simulink model "MIL4L3_SW6_V1_20220211"  (R2018b)
settings: Solver=FixedStepAuto  StartTime=0.0  StopTime=inf  FixedStep=0.001  RelTol=1e-3
PreLoadFcn:
  | A0_MILtest;
undefined symbols (not defined in the file or in its folder): Clb_ICADirect_LaneDisp_StateFive, Clb_ICADirect_LaneDisp_StateFour, Clb_ICADirect_LaneDisp_StateOne, Clb_ICADirect_LaneDisp_StateThree, Clb_ICADirect_LaneDisp_StateTwo, Clb_ICADirect_LaneDisp_StateZero, Clb_ICADirect_LaneDispSW, Clb_ICADirect_TrnLghtsCom_Switch, Clb_ICADirect_TrnLghtsCom_Value, Clb_ICADirect_TrnLghtsCrtl_Inhb, IMAP_Clb_ACU_Driver_Belt, IMAP_Clb_ACU_Driver_Belt_Over, IMAP_Clb_ACU_Passenger_Belt, IMAP_Clb_ACU_Passenger_Belt_Over, IMAP_Clb_ACU_RearLeft_Belt, IMAP_Clb_ACU_RearLeft_Belt_Over, IMAP_Clb_ACU_RearMiddle_Belt, IMAP_Clb_ACU_RearMiddle_Belt_Over, IMAP_Clb_ACU_RearRight_Belt, IMAP_Clb_ACU_RearRight_Belt_Over, IMAP_Clb_AEB_Switch, IMAP_Clb_AEB_Switch_Over, IMAP_Clb_ALC_TLC_Mode, IMAP_Clb_ALC_TLC_Mode_Over, IMAP_Clb_BCM_Battery_Voltage, IMAP_Clb_BCM_Battery_Voltage_Over, IMAP_Clb_BCM_BrakeLamp_State, IMAP_Clb_BCM_BrakeLamp_State_Over, IMAP_Clb_BCM_CHMSL_Status, IMAP_Clb_BCM_CHMSL_Status_Over, IMAP_Clb_BCM_Door_Lock_State, IMAP_Clb_BCM_Door_Lock_State_Over, IMAP_Clb_BCM_FrontWiper_State, IMAP_Clb_BCM_FrontWiper_State_Over, IMAP_Clb_BCM_FrontWiper_Switch, IMAP_Clb_BCM_FrontWiper_Switch_Over, IMAP_Clb_BCM_HazardLamp, IMAP_Clb_BCM_HazardLamp_Over, IMAP_Clb_BCM_HazardLamp_Switch, IMAP_Clb_BCM_HazardLamp_Switch_Over, IMAP_Clb_BCM_HighBeam_State, IMAP_Clb_BCM_HighBeam_State_Over, IMAP_Clb_BCM_Ignition_State, IMAP_Clb_BCM_Ignition_State_Over, IMAP_Clb_BCM_IHBC_Enabled, IMAP_Clb_BCM_IHBC_Enabled_Over, IMAP_Clb_BCM_Left_Light, IMAP_Clb_BCM_Left_Light_Over, IMAP_Clb_BCM_LeftTurn_Switch, IMAP_Clb_BCM_LeftTurn_Switch_Over, IMAP_Clb_BCM_LF_Door_State, IMAP_Clb_BCM_LF_Door_State_Over, IMAP_Clb_BCM_LowBeam_State, IMAP_Clb_BCM_LowBeam_State_Over, IMAP_Clb_BCM_LR_Door_State, IMAP_Clb_BCM_LR_Door_State_Over, IMAP_Clb_BCM_RF_Door_State, IMAP_Clb_BCM_RF_Door_State_Over, IMAP_Clb_BCM_Right_Light, IMAP_Clb_BCM_Right_Light_Over ... (+547)
libraries: CarMaker4SL x2153, simulink x292, dspstat3 x3, canmsglib x2, simulink_extras x1
(part 19 of 52)

== system MIL4L3_SW6_V1_20220211/CarMaker/VehicleControl/Traffic Attribution Define1/T17 ==
  Define CM Dict 0 : CarMaker4SL/Define CM Dict  xname=User.IO.Out.T17.ExistenceProbability  xmono=off  xtype=Double4  xdvaplace=IO_Out  xnstates=0  xfirststate=0  xinitial=0.95
  Define CM Dict 1 : CarMaker4SL/Define CM Dict  xname=User.IO.Out.T17.class  xmono=off  xtype=Double4  xdvaplace=IO_Out  xnstates=0  xfirststate=0  xinitial=1
  Define CM Dict 2 : CarMaker4SL/Define CM Dict  xname=User.IO.Out.T17.ObjectInfo  xmono=off  xtype=Double4  xdvaplace=IO_Out  xnstates=0  xfirststate=0  xinitial=2
  Define CM Dict 3 : CarMaker4SL/Define CM Dict  xname=User.IO.Out.T17.ClassHighestProb  xmono=off  xtype=Double4  xdvaplace=IO_Out  xnstates=0  xfirststate=0  xinitial=2
  Define CM Dict 4 : CarMaker4SL/Define CM Dict  xname=User.IO.Out.T17.status  xmono=off  xtype=Double4  xdvaplace=IO_Out  xnstates=0  xfirststate=0  xinitial=0
  Define CM Dict 5 : CarMaker4SL/Define CM Dict  xname=User.IO.Out.T17.probility  xmono=off  xtype=Double4  xdvaplace=IO_Out  xnstates=0  xfirststate=0  xinitial=0.9
  Define CM Dict 6 : CarMaker4SL/Define CM Dict  xname=User.IO.Out.T17.power  xmono=off  xtype=Double4  xdvaplace=IO_Out  xnstates=0  xfirststate=0  xinitial=90
  Define CM Dict 7 : CarMaker4SL/Define CM Dict  xname=User.IO.Out.T17.Turn_signal  xmono=off  xtype=Double4  xdvaplace=IO_Out  xnstates=0  xfirststate=0  xinitial=0
  Define CM Dict 8 : CarMaker4SL/Define CM Dict  xname=User.IO.Out.T17.BrakeLight  xmono=off  xtype=Double4  xdvaplace=IO_Out  xnstates=0  xfirststate=0  xinitial=0
  Define CM Dict5 : CarMaker4SL/Define CM Dict  xname=User.IO.Out.T17.longdistance  xmono=off  xtype=Double4  xdvaplace=None  xnstates=0  xfirststate=0  xinitial=0
  Define CM Dict6 : CarMaker4SL/Define CM Dict  xname=User.IO.Out.T17.RelVxValid  xmono=off  xtype=Double4  xdvaplace=None  xnstates=0  xfirststate=0  xinitial=1
  Define CM Dict7 : CarMaker4SL/Define CM Dict  xname=User.IO.Out.T17.RelVyValid  xmono=off  xtype=Double4  xdvaplace=None  xnstates=0  xfirststate=0  xinitial=1
  Define CM Dict8 : CarMaker4SL/Define CM Dict  xname=User.IO.Out.T17.TypeProb  xmono=off  xtype=Double4  xdvaplace=None  xnstates=0  xfirststate=0  xinitial=1
  Define CM Dict9 : CarMaker4SL/Define CM Dict  xname=User.IO.Out.T17.Measured  xmono=off  xtype=Double4  xdvaplace=None  xnstates=0  xfirststate=0  xinitial=2

== system MIL4L3_SW6_V1_20220211/CarMaker/VehicleControl/Traffic Attribution Define1/T18 ==
  Define CM Dict 0 : CarMaker4SL/Define CM Dict  xname=User.IO.Out.T18.ExistenceProbability  xmono=off  xtype=Double4  xdvaplace=IO_Out  xnstates=0  xfirststate=0  xinitial=0.95
  Define CM Dict 1 : CarMaker4SL/Define CM Dict  xname=User.IO.Out.T18.class  xmono=off  xtype=Double4  xdvaplace=IO_Out  xnstates=0  xfirststate=0  xinitial=1
  Define CM Dict 2 : CarMaker4SL/Define CM Dict  xname=User.IO.Out.T18.ObjectInfo  xmono=off  xtype=Double4  xdvaplace=IO_Out  xnstates=0  xfirststate=0  xinitial=2
  Define CM Dict 3 : CarMaker4SL/Define CM Dict  xname=User.IO.Out.T18.ClassHighestProb  xmono=off  xtype=Double4  xdvaplace=IO_Out  xnstates=0  xfirststate=0  xinitial=2
  Define CM Dict 4 : CarMaker4SL/Define CM Dict  xname=User.IO.Out.T18.status  xmono=off  xtype=Double4  xdvaplace=IO_Out  xnstates=0  xfirststate=0  xinitial=0
  Define CM Dict 5 : CarMaker4SL/Define CM Dict  xname=User.IO.Out.T18.probility  xmono=off  xtype=Double4  xdvaplace=IO_Out  xnstates=0  xfirststate=0  xinitial=0.9
  Define CM Dict 6 : CarMaker4SL/Define CM Dict  xname=User.IO.Out.T18.power  xmono=off  xtype=Double4  xdvaplace=IO_Out  xnstates=0  xfirststate=0  xinitial=90
  Define CM Dict 7 : CarMaker4SL/Define CM Dict  xname=User.IO.Out.T18.Turn_signal  xmono=off  xtype=Double4  xdvaplace=IO_Out  xnstates=0  xfirststate=0  xinitial=0
  Define CM Dict 8 : CarMaker4SL/Define CM Dict  xname=User.IO.Out.T18.BrakeLight  xmono=off  xtype=Double4  xdvaplace=IO_Out  xnstates=0  xfirststate=0  xinitial=0
  Define CM Dict5 : CarMaker4SL/Define CM Dict  xname=User.IO.Out.T18.longdistance  xmono=off  xtype=Double4  xdvaplace=None  xnstates=0  xfirststate=0  xinitial=0
  Define CM Dict6 : CarMaker4SL/Define CM Dict  xname=User.IO.Out.T18.RelVxValid  xmono=off  xtype=Double4  xdvaplace=None  xnstates=0  xfirststate=0  xinitial=1
  Define CM Dict7 : CarMaker4SL/Define CM Dict  xname=User.IO.Out.T18.RelVyValid  xmono=off  xtype=Double4  xdvaplace=None  xnstates=0  xfirststate=0  xinitial=1
  Define CM Dict8 : CarMaker4SL/Define CM Dict  xname=User.IO.Out.T18.TypeProb  xmono=off  xtype=Double4  xdvaplace=None  xnstates=0  xfirststate=0  xinitial=1
  Define CM Dict9 : CarMaker4SL/Define CM Dict  xname=User.IO.Out.T18.Measured  xmono=off  xtype=Double4  xdvaplace=None  xnstates=0  xfirststate=0  xinitial=2

== system MIL4L3_SW6_V1_20220211/CarMaker/VehicleControl/Traffic Attribution Define1/T19 ==
  Define CM Dict 0 : CarMaker4SL/Define CM Dict  xname=User.IO.Out.T19.ExistenceProbability  xmono=off  xtype=Double4  xdvaplace=IO_Out  xnstates=0  xfirststate=0  xinitial=0.95
  Define CM Dict 1 : CarMaker4SL/Define CM Dict  xname=User.IO.Out.T19.class  xmono=off  xtype=Double4  xdvaplace=IO_Out  xnstates=0  xfirststate=0  xinitial=1
  Define CM Dict 2 : CarMaker4SL/Define CM Dict  xname=User.IO.Out.T19.ObjectInfo  xmono=off  xtype=Double4  xdvaplace=IO_Out  xnstates=0  xfirststate=0  xinitial=2
  Define CM Dict 3 : CarMaker4SL/Define CM Dict  xname=User.IO.Out.T19.ClassHighestProb  xmono=off  xtype=Double4  xdvaplace=IO_Out  xnstates=0  xfirststate=0  xinitial=2
  Define CM Dict 4 : CarMaker4SL/Define CM Dict  xname=User.IO.Out.T19.status  xmono=off  xtype=Double4  xdvaplace=IO_Out  xnstates=0  xfirststate=0  xinitial=0
  Define CM Dict 5 : CarMaker4SL/Define CM Dict  xname=User.IO.Out.T19.probility  xmono=off  xtype=Double4  xdvaplace=IO_Out  xnstates=0  xfirststate=0  xinitial=0.9
  Define CM Dict 6 : CarMaker4SL/Define CM Dict  xname=User.IO.Out.T19.power  xmono=off  xtype=Double4  xdvaplace=IO_Out  xnstates=0  xfirststate=0  xinitial=90
  Define CM Dict 7 : CarMaker4SL/Define CM Dict  xname=User.IO.Out.T19.Turn_signal  xmono=off  xtype=Double4  xdvaplace=IO_Out  xnstates=0  xfirststate=0  xinitial=0
  Define CM Dict 8 : CarMaker4SL/Define CM Dict  xname=User.IO.Out.T19.BrakeLight  xmono=off  xtype=Double4  xdvaplace=IO_Out  xnstates=0  xfirststate=0  xinitial=0
  Define CM Dict5 : CarMaker4SL/Define CM Dict  xname=User.IO.Out.T19.longdistance  xmono=off  xtype=Double4  xdvaplace=None  xnstates=0  xfirststate=0  xinitial=0
  Define CM Dict6 : CarMaker4SL/Define CM Dict  xname=User.IO.Out.T19.RelVxValid  xmono=off  xtype=Double4  xdvaplace=None  xnstates=0  xfirststate=0  xinitial=1
  Define CM Dict7 : CarMaker4SL/Define CM Dict  xname=User.IO.Out.T19.RelVyValid  xmono=off  xtype=Double4  xdvaplace=None  xnstates=0  xfirststate=0  xinitial=1
  Define CM Dict8 : CarMaker4SL/Define CM Dict  xname=User.IO.Out.T19.TypeProb  xmono=off  xtype=Double4  xdvaplace=None  xnstates=0  xfirststate=0  xinitial=1
  Define CM Dict9 : CarMaker4SL/Define CM Dict  xname=User.IO.Out.T19.Measured  xmono=off  xtype=Double4  xdvaplace=None  xnstates=0  xfirststate=0  xinitial=2

== system MIL4L3_SW6_V1_20220211/CarMaker/VehicleControl/Traffic Attribution Define1/T20 ==
  Define CM Dict 0 : CarMaker4SL/Define CM Dict  xname=User.IO.Out.T20.ExistenceProbability  xmono=off  xtype=Double4  xdvaplace=IO_Out  xnstates=0  xfirststate=0  xinitial=0.95
  Define CM Dict 1 : CarMaker4SL/Define CM Dict  xname=User.IO.Out.T20.class  xmono=off  xtype=Double4  xdvaplace=IO_Out  xnstates=0  xfirststate=0  xinitial=1
  Define CM Dict 2 : CarMaker4SL/Define CM Dict  xname=User.IO.Out.T20.ObjectInfo  xmono=off  xtype=Double4  xdvaplace=IO_Out  xnstates=0  xfirststate=0  xinitial=2
  Define CM Dict 3 : CarMaker4SL/Define CM Dict  xname=User.IO.Out.T20.ClassHighestProb  xmono=off  xtype=Double4  xdvaplace=IO_Out  xnstates=0  xfirststate=0  xinitial=2
  Define CM Dict 4 : CarMaker4SL/Define CM Dict  xname=User.IO.Out.T20.status  xmono=off  xtype=Double4  xdvaplace=IO_Out  xnstates=0  xfirststate=0  xinitial=0
  Define CM Dict 5 : CarMaker4SL/Define CM Dict  xname=User.IO.Out.T20.probility  xmono=off  xtype=Double4  xdvaplace=IO_Out  xnstates=0  xfirststate=0  xinitial=0.9
  Define CM Dict 6 : CarMaker4SL/Define CM Dict  xname=User.IO.Out.T20.power  xmono=off  xtype=Double4  xdvaplace=IO_Out  xnstates=0  xfirststate=0  xinitial=90
  Define CM Dict 7 : CarMaker4SL/Define CM Dict  xname=User.IO.Out.T20.Turn_signal  xmono=off  xtype=Double4  xdvaplace=IO_Out  xnstates=0  xfirststate=0  xinitial=0
  Define CM Dict 8 : CarMaker4SL/Define CM Dict  xname=User.IO.Out.T20.BrakeLight  xmono=off  xtype=Double4  xdvaplace=IO_Out  xnstates=0  xfirststate=0  xinitial=0
  Define CM Dict5 : CarMaker4SL/Define CM Dict  xname=User.IO.Out.T20.longdistance  xmono=off  xtype=Double4  xdvaplace=None  xnstates=0  xfirststate=0  xinitial=0
  Define CM Dict6 : CarMaker4SL/Define CM Dict  xname=User.IO.Out.T20.RelVxValid  xmono=off  xtype=Double4  xdvaplace=None  xnstates=0  xfirststate=0  xinitial=1
  Define CM Dict7 : CarMaker4SL/Define CM Dict  xname=User.IO.Out.T20.RelVyValid  xmono=off  xtype=Double4  xdvaplace=None  xnstates=0  xfirststate=0  xinitial=1
  Define CM Dict8 : CarMaker4SL/Define CM Dict  xname=User.IO.Out.T20.TypeProb  xmono=off  xtype=Double4  xdvaplace=None  xnstates=0  xfirststate=0  xinitial=1
  Define CM Dict9 : CarMaker4SL/Define CM Dict  xname=User.IO.Out.T20.Measured  xmono=off  xtype=Double4  xdvaplace=None  xnstates=0  xfirststate=0  xinitial=2

== system MIL4L3_SW6_V1_20220211/CarMaker/VehicleControl/Traffic Attribution Define1/T21 ==
  Define CM Dict 0 : CarMaker4SL/Define CM Dict  xname=User.IO.Out.T21.ExistenceProbability  xmono=off  xtype=Double4  xdvaplace=IO_Out  xnstates=0  xfirststate=0  xinitial=0.95
  Define CM Dict 1 : CarMaker4SL/Define CM Dict  xname=User.IO.Out.T21.class  xmono=off  xtype=Double4  xdvaplace=IO_Out  xnstates=0  xfirststate=0  xinitial=1
  Define CM Dict 2 : CarMaker4SL/Define CM Dict  xname=User.IO.Out.T21.ObjectInfo  xmono=off  xtype=Double4  xdvaplace=IO_Out  xnstates=0  xfirststate=0  xinitial=2
  Define CM Dict 3 : CarMaker4SL/Define CM Dict  xname=User.IO.Out.T21.ClassHighestProb  xmono=off  xtype=Double4  xdvaplace=IO_Out  xnstates=0  xfirststate=0  xinitial=2
  Define CM Dict 4 : CarMaker4SL/Define CM Dict  xname=User.IO.Out.T21.status  xmono=off  xtype=Double4  xdvaplace=IO_Out  xnstates=0  xfirststate=0  xinitial=0
  Define CM Dict 5 : CarMaker4SL/Define CM Dict  xname=User.IO.Out.T21.probility  xmono=off  xtype=Double4  xdvaplace=IO_Out  xnstates=0  xfirststate=0  xinitial=0.9
  Define CM Dict 6 : CarMaker4SL/Define CM Dict  xname=User.IO.Out.T21.power  xmono=off  xtype=Double4  xdvaplace=IO_Out  xnstates=0  xfirststate=0  xinitial=90
  Define CM Dict 7 : CarMaker4SL/Define CM Dict  xname=User.IO.Out.T21.Turn_signal  xmono=off  xtype=Double4  xdvaplace=IO_Out  xnstates=0  xfirststate=0  xinitial=0
  Define CM Dict 8 : CarMaker4SL/Define CM Dict  xname=User.IO.Out.T21.BrakeLight  xmono=off  xtype=Double4  xdvaplace=IO_Out  xnstates=0  xfirststate=0  xinitial=0
  Define CM Dict5 : CarMaker4SL/Define CM Dict  xname=User.IO.Out.T21.longdistance  xmono=off  xtype=Double4  xdvaplace=None  xnstates=0  xfirststate=0  xinitial=0
  Define CM Dict6 : CarMaker4SL/Define CM Dict  xname=User.IO.Out.T21.RelVxValid  xmono=off  xtype=Double4  xdvaplace=None  xnstates=0  xfirststate=0  xinitial=1
  Define CM Dict7 : CarMaker4SL/Define CM Dict  xname=User.IO.Out.T21.RelVyValid  xmono=off  xtype=Double4  xdvaplace=None  xnstates=0  xfirststate=0  xinitial=1
  Define CM Dict8 : CarMaker4SL/Define CM Dict  xname=User.IO.Out.T21.TypeProb  xmono=off  xtype=Double4  xdvaplace=None  xnstates=0  xfirststate=0  xinitial=1
  Define CM Dict9 : CarMaker4SL/Define CM Dict  xname=User.IO.Out.T21.Measured  xmono=off  xtype=Double4  xdvaplace=None  xnstates=0  xfirststate=0  xinitial=2

== system MIL4L3_SW6_V1_20220211/CarMaker/VehicleControl/Traffic Attribution Define1/T22 ==
  Define CM Dict 0 : CarMaker4SL/Define CM Dict  xname=User.IO.Out.T22.ExistenceProbability  xmono=off  xtype=Double4  xdvaplace=IO_Out  xnstates=0  xfirststate=0  xinitial=0.95
  Define CM Dict 1 : CarMaker4SL/Define CM Dict  xname=User.IO.Out.T22.class  xmono=off  xtype=Double4  xdvaplace=IO_Out  xnstates=0  xfirststate=0  xinitial=1
  Define CM Dict 2 : CarMaker4SL/Define CM Dict  xname=User.IO.Out.T22.ObjectInfo  xmono=off  xtype=Double4  xdvaplace=IO_Out  xnstates=0  xfirststate=0  xinitial=2
  Define CM Dict 3 : CarMaker4SL/Define CM Dict  xname=User.IO.Out.T22.ClassHighestProb  xmono=off  xtype=Double4  xdvaplace=IO_Out  xnstates=0  xfirststate=0  xinitial=2
  Define CM Dict 4 : CarMaker4SL/Define CM Dict  xname=User.IO.Out.T22.status  xmono=off  xtype=Double4  xdvaplace=IO_Out  xnstates=0  xfirststate=0  xinitial=0
  Define CM Dict 5 : CarMaker4SL/Define CM Dict  xname=User.IO.Out.T22.probility  xmono=off  xtype=Double4  xdvaplace=IO_Out  xnstates=0  xfirststate=0  xinitial=0.9
  Define CM Dict 6 : CarMaker4SL/Define CM Dict  xname=User.IO.Out.T22.power  xmono=off  xtype=Double4  xdvaplace=IO_Out  xnstates=0  xfirststate=0  xinitial=90
  Define CM Dict 7 : CarMaker4SL/Define CM Dict  xname=User.IO.Out.T22.Turn_signal  xmono=off  xtype=Double4  xdvaplace=IO_Out  xnstates=0  xfirststate=0  xinitial=0
  Define CM Dict 8 : CarMaker4SL/Define CM Dict  xname=User.IO.Out.T22.BrakeLight  xmono=off  xtype=Double4  xdvaplace=IO_Out  xnstates=0  xfirststate=0  xinitial=0
  Define CM Dict5 : CarMaker4SL/Define CM Dict  xname=User.IO.Out.T22.longdistance  xmono=off  xtype=Double4  xdvaplace=None  xnstates=0  xfirststate=0  xinitial=0
  Define CM Dict6 : CarMaker4SL/Define CM Dict  xname=User.IO.Out.T22.RelVxValid  xmono=off  xtype=Double4  xdvaplace=None  xnstates=0  xfirststate=0  xinitial=1
  Define CM Dict7 : CarMaker4SL/Define CM Dict  xname=User.IO.Out.T22.RelVyValid  xmono=off  xtype=Double4  xdvaplace=None  xnstates=0  xfirststate=0  xinitial=1
  Define CM Dict8 : CarMaker4SL/Define CM Dict  xname=User.IO.Out.T22.TypeProb  xmono=off  xtype=Double4  xdvaplace=None  xnstates=0  xfirststate=0  xinitial=1
  Define CM Dict9 : CarMaker4SL/Define CM Dict  xname=User.IO.Out.T22.Measured  xmono=off  xtype=Double4  xdvaplace=None  xnstates=0  xfirststate=0  xinitial=2

== system MIL4L3_SW6_V1_20220211/CarMaker/VehicleControl/Traffic Attribution Define1/T23 ==
  Define CM Dict 0 : CarMaker4SL/Define CM Dict  xname=User.IO.Out.T23.ExistenceProbability  xmono=off  xtype=Double4  xdvaplace=IO_Out  xnstates=0  xfirststate=0  xinitial=0.95
  Define CM Dict 1 : CarMaker4SL/Define CM Dict  xname=User.IO.Out.T23.class  xmono=off  xtype=Double4  xdvaplace=IO_Out  xnstates=0  xfirststate=0  xinitial=1
  Define CM Dict 2 : CarMaker4SL/Define CM Dict  xname=User.IO.Out.T23.ObjectInfo  xmono=off  xtype=Double4  xdvaplace=IO_Out  xnstates=0  xfirststate=0  xinitial=2
  Define CM Dict 3 : CarMaker4SL/Define CM Dict  xname=User.IO.Out.T23.ClassHighestProb  xmono=off  xtype=Double4  xdvaplace=IO_Out  xnstates=0  xfirststate=0  xinitial=2
  Define CM Dict 4 : CarMaker4SL/Define CM Dict  xname=User.IO.Out.T23.status  xmono=off  xtype=Double4  xdvaplace=IO_Out  xnstates=0  xfirststate=0  xinitial=0
  Define CM Dict 5 : CarMaker4SL/Define CM Dict  xname=User.IO.Out.T23.probility  xmono=off  xtype=Double4  xdvaplace=IO_Out  xnstates=0  xfirststate=0  xinitial=0.9
  Define CM Dict 6 : CarMaker4SL/Define CM Dict  xname=User.IO.Out.T23.power  xmono=off  xtype=Double4  xdvaplace=IO_Out  xnstates=0  xfirststate=0  xinitial=90
  Define CM Dict 7 : CarMaker4SL/Define CM Dict  xname=User.IO.Out.T23.Turn_signal  xmono=off  xtype=Double4  xdvaplace=IO_Out  xnstates=0  xfirststate=0  xinitial=0
  Define CM Dict 8 : CarMaker4SL/Define CM Dict  xname=User.IO.Out.T23.BrakeLight  xmono=off  xtype=Double4  xdvaplace=IO_Out  xnstates=0  xfirststate=0  xinitial=0
  Define CM Dict5 : CarMaker4SL/Define CM Dict  xname=User.IO.Out.T23.longdistance  xmono=off  xtype=Double4  xdvaplace=None  xnstates=0  xfirststate=0  xinitial=0
  Define CM Dict6 : CarMaker4SL/Define CM Dict  xname=User.IO.Out.T23.RelVxValid  xmono=off  xtype=Double4  xdvaplace=None  xnstates=0  xfirststate=0  xinitial=1
  Define CM Dict7 : CarMaker4SL/Define CM Dict  xname=User.IO.Out.T23.RelVyValid  xmono=off  xtype=Double4  xdvaplace=None  xnstates=0  xfirststate=0  xinitial=1
  Define CM Dict8 : CarMaker4SL/Define CM Dict  xname=User.IO.Out.T23.TypeProb  xmono=off  xtype=Double4  xdvaplace=None  xnstates=0  xfirststate=0  xinitial=1
  Define CM Dict9 : CarMaker4SL/Define CM Dict  xname=User.IO.Out.T23.Measured  xmono=off  xtype=Double4  xdvaplace=None  xnstates=0  xfirststate=0  xinitial=2

== system MIL4L3_SW6_V1_20220211/CarMaker/VehicleControl/User.IO.Out/ActuatorStatus2Ctrl ==
  BusCreator : BusCreator  Inputs=38
  Read CM Dict : CarMaker4SL/Read CM Dict  xname=User.IO.Out.EPS_LKAState  xsync=off
  Read CM Dict1 : CarMaker4SL/Read CM Dict  xname=User.IO.Out.EPSErrSt  xsync=off
  Read CM Dict10 : CarMaker4SL/Read CM Dict  xname=User.IO.Out.BCM_RRDoorSt  xsync=off
  Read CM Dict11 : CarMaker4SL/Read CM Dict  xname=User.IO.Out.BCM_LRDoorSt  xsync=off
  Read CM Dict12 : CarMaker4SL/Read CM Dict  xname=User.IO.Out.BCM_DoorLockSt  xsync=off
  Read CM Dict13 : CarMaker4SL/Read CM Dict  xname=User.IO.Out.EMS_Status_ACC  xsync=off
  Read CM Dict14 : CarMaker4SL/Read CM Dict  xname=User.IO.Out.SCC_LeftSwSig  xsync=off
  Read CM Dict15 : CarMaker4SL/Read CM Dict  xname=User.IO.Out.SCC_RightSwSig  xsync=off
  Read CM Dict16 : CarMaker4SL/Read CM Dict  xname=User.IO.Out.GW_EMS_AccPedFlt  xsync=off
  Read CM Dict17 : CarMaker4SL/Read CM Dict  xname=User.IO.Out.BCM_IgnitionSt  xsync=off
  Read CM Dict18 : CarMaker4SL/Read CM Dict  xname=User.IO.Out.EMS_AccPedalR  xsync=off
  Read CM Dict19 : CarMaker4SL/Read CM Dict  xname=User.IO.Out.GW_EMS_AccPedal  xsync=off
  Read CM Dict2 : CarMaker4SL/Read CM Dict  xname=User.IO.Out.BCM_HazardLampSt  xsync=off
  Read CM Dict20 : CarMaker4SL/Read CM Dict  xname=User.IO.Out.ACU_DriverBelt  xsync=off
  Read CM Dict21 : CarMaker4SL/Read CM Dict  xname=User.IO.Out.Brake_pedalFault  xsync=off
  Read CM Dict22 : CarMaker4SL/Read CM Dict  xname=User.IO.Out.GW_TCU_ATFailure  xsync=off
  Read CM Dict23 : CarMaker4SL/Read CM Dict  xname=User.IO.Out.ESC_ESCOFF  xsync=off
  Read CM Dict24 : CarMaker4SL/Read CM Dict  xname=User.IO.Out.GW_Speed_Lim_On  xsync=off
  Read CM Dict25 : CarMaker4SL/Read CM Dict  xname=User.IO.Out.BCM_FrontWiperSt  xsync=off
  Read CM Dict26 : CarMaker4SL/Read CM Dict  xname=User.IO.Out.ACU_PassengerBelt  xsync=off
  Read CM Dict27 : CarMaker4SL/Read CM Dict  xname=User.IO.Out.GW_EMS_EngStatus  xsync=off
  Read CM Dict28 : CarMaker4SL/Read CM Dict  xname=User.IO.Out.ESC_AEB_Status  xsync=off
  Read CM Dict29 : CarMaker4SL/Read CM Dict  xname=User.IO.Out.ESC_AEB_Available  xsync=off
  Read CM Dict3 : CarMaker4SL/Read CM Dict  xname=User.IO.Out.BCM_LetfligthSt  xsync=off
  Read CM Dict30 : CarMaker4SL/Read CM Dict  xname=User.IO.Out.ESC_ACC_Status  xsync=off
  Read CM Dict31 : CarMaker4SL/Read CM Dict  xname=User.IO.Out.ESC_ACC_Available  xsync=off
  Read CM Dict32 : CarMaker4SL/Read CM Dict  xname=User.IO.Out.EMS_ACCctlAvail  xsync=off
  Read CM Dict33 : CarMaker4SL/Read CM Dict  xname=User.IO.Out.EMS_ACC_Ihibited  xsync=off
  Read CM Dict34 : CarMaker4SL/Read CM Dict  xname=User.IO.Out.EPB_EPBStatus  xsync=off
  Read CM Dict35 : CarMaker4SL/Read CM Dict  xname=User.IO.Out.EPS_SteerHoldSt  xsync=off
  Read CM Dict36 : CarMaker4SL/Read CM Dict  xname=User.IO.Out.BCM_BattVolt  xsync=off
  Read CM Dict37 : CarMaker4SL/Read CM Dict  xname=User.IO.Out.ICAD_DecionState  xsync=off
  Read CM Dict4 : CarMaker4SL/Read CM Dict  xname=User.IO.Out.BCM_RightligthSt  xsync=off
  Read CM Dict5 : CarMaker4SL/Read CM Dict  xname=User.IO.Out.ESC_BLRequest  xsync=off
  Read CM Dict6 : CarMaker4SL/Read CM Dict  xname=User.IO.Out.BCM_Openingstates  xsync=off
  Read CM Dict7 : CarMaker4SL/Read CM Dict  xname=User.IO.Out.BCM_TrunkSt  xsync=off
  Read CM Dict8 : CarMaker4SL/Read CM Dict  xname=User.IO.Out.BCM_LFDoorSt  xsync=off
  Read CM Dict9 : CarMaker4SL/Read CM Dict  xname=User.IO.Out.BCM_RFDoorSt  xsync=off
  tag scope: ActuatorStatus2Ctrl=global
  wires:
  Read CM Dict6/1 -> BusCreator/7  "User.IO.Out.BCM_Openingstates"
  Read CM Dict7/1 -> BusCreator/8  "User.IO.Out.BCM_TrunkSt"
  Read CM Dict8/1 -> BusCreator/9  "User.IO.Out.BCM_LFDoorSt"
  Read CM Dict9/1 -> BusCreator/10  "User.IO.Out.BCM_RFDoorSt"
  Read CM Dict10/1 -> BusCreator/11  "User.IO.Out.BCM_RRDoorSt"
  Read CM Dict11/1 -> BusCreator/12  "User.IO.Out.BCM_LRDoorSt"
  Read CM Dict4/1 -> BusCreator/5  "User.IO.Out.BCM_RightligthSt"
  Read CM Dict5/1 -> BusCreator/6  "User.IO.Out.ESC_BLRequest"
  Read CM Dict14/1 -> BusCreator/13  "User.IO.Out.SCC_LeftSwSig"
  Read CM Dict15/1 -> BusCreator/14  "User.IO.Out.SCC_RightSwSig"
  Read CM Dict/1 -> BusCreator/1  "User.IO.Out.EPS_LKAState"
  Read CM Dict1/1 -> BusCreator/2  "User.IO.Out.EPSErrSt"
  Read CM Dict2/1 -> BusCreator/3  "User.IO.Out.BCM_HazardLampSt"
  Read CM Dict3/1 -> BusCreator/4  "User.IO.Out.BCM_LetfligthSt"
  Read CM Dict12/1 -> BusCreator/15  "User.IO.Out.BCM_DoorLockSt"
  Read CM Dict13/1 -> BusCreator/16  "User.IO.Out.EMS_Status_ACC"
  Read CM Dict18/1 -> BusCreator/17  "User.IO.Out.EMS_AccPedalR"
  Read CM Dict19/1 -> BusCreator/18  "User.IO.Out.GW_EMS_AccPedal"
  Read CM Dict16/1 -> BusCreator/19  "User.IO.Out.GW_EMS_AccPedFlt"
  Read CM Dict17/1 -> BusCreator/20  "User.IO.Out.BCM_IgnitionSt"
  Read CM Dict20/1 -> BusCreator/21  "User.IO.Out.ACU_DriverBelt"
  Read CM Dict23/1 -> BusCreator/22  "User.IO.Out.ESC_ESCOFF"
  Read CM Dict24/1 -> BusCreator/23  "User.IO.Out.GW_Speed_Lim_On"
  Read CM Dict21/1 -> BusCreator/24  "User.IO.Out.Brake_pedalFault"
  Read CM Dict22/1 -> BusCreator/25  "User.IO.Out.GW_TCU_ATFailure"
  Read CM Dict29/1 -> BusCreator/28  "User.IO.Out.ESC_AEB_Available"
  Read CM Dict30/1 -> BusCreator/29  "User.IO.Out.ESC_ACC_Status"
  Read CM Dict31/1 -> BusCreator/30  "User.IO.Out.ESC_ACC_Available"
  Read CM Dict26/1 -> BusCreator/32  "User.IO.Out.ACU_PassengerBelt"
  Read CM Dict32/1 -> BusCreator/33  "User.IO.Out.EMS_ACCctlAvail"
  Read CM Dict33/1 -> BusCreator/34  "User.IO.Out.EMS_ACC_Ihibited"
  Read CM Dict27/1 -> BusCreator/26  "User.IO.Out.GW_EMS_EngStatus"
  Read CM Dict28/1 -> BusCreator/27  "User.IO.Out.ESC_AEB_Status"
  Read CM Dict25/1 -> BusCreator/31  "User.IO.Out.BCM_FrontWiperSt"
  Read CM Dict35/1 -> BusCreator/36  "User.IO.Out.EPS_SteerHoldSt"
  Read CM Dict36/1 -> BusCreator/37  "User.IO.Out.BCM_BattVolt"
  Read CM Dict34/1 -> BusCreator/35  "User.IO.Out.EPB_EPBStatus"
  Read CM Dict37/1 -> BusCreator/38  "User.IO.Out.ICAD_DecionState"
  BusCreator/1 -> [ActuatorStatus2Ctrl]

== system MIL4L3_SW6_V1_20220211/CarMaker/VehicleControl/User.IO.Out/MP5_Cmd2Ctrl ==
  BusCreator : BusCreator  Inputs=27
  Read CM Dict : CarMaker4SL/Read CM Dict  xname=User.IO.Out.Mp5_LKA_main_SW  xsync=off
  Read CM Dict1 : CarMaker4SL/Read CM Dict  xname=User.IO.Out.Mp5_LKA_Mode  xsync=off
  Read CM Dict10 : CarMaker4SL/Read CM Dict  xname=User.IO.Out.MP5_ALCTLC_Mode  xsync=off
  Read CM Dict11 : CarMaker4SL/Read CM Dict  xname=User.IO.Out.Mp5_ESA_Cfg  xsync=off
  Read CM Dict12 : CarMaker4SL/Read CM Dict  xname=User.IO.Out.Mp5_ELK_Cfg  xsync=off
  Read CM Dict13 : CarMaker4SL/Read CM Dict  xname=User.IO.Out.AutoParkingCmd  xsync=off
  Read CM Dict14 : CarMaker4SL/Read CM Dict  xname=User.IO.Out.PEPS_RKECommand  xsync=off
  Read CM Dict15 : CarMaker4SL/Read CM Dict  xname=User.IO.Out.MP5_BSD_LCW_ACT  xsync=off
  Read CM Dict16 : CarMaker4SL/Read CM Dict  xname=User.IO.Out.MP5_RCTA_ACT  xsync=off
  Read CM Dict17 : CarMaker4SL/Read CM Dict  xname=User.IO.Out.MP5_DOW_ACT  xsync=off
  Read CM Dict18 : CarMaker4SL/Read CM Dict  xname=User.IO.Out.JaBrakConf  xsync=off
  Read CM Dict19 : CarMaker4SL/Read CM Dict  xname=User.IO.Out.JaAlertConf  xsync=off
  Read CM Dict2 : CarMaker4SL/Read CM Dict  xname=User.IO.Out.MP5_AEBSwitch  xsync=off
  Read CM Dict20 : CarMaker4SL/Read CM Dict  xname=User.IO.Out.JaAlertSens  xsync=off
  Read CM Dict21 : CarMaker4SL/Read CM Dict  xname=User.IO.Out.LFConf  xsync=off
  Read CM Dict22 : CarMaker4SL/Read CM Dict  xname=User.IO.Out.MP5_FCTA_ACT  xsync=off
  Read CM Dict23 : CarMaker4SL/Read CM Dict  xname=User.IO.Out.ICAConf  xsync=off
  Read CM Dict24 : CarMaker4SL/Read CM Dict  xname=User.IO.Out.AlcSens  xsync=off
  Read CM Dict25 : CarMaker4SL/Read CM Dict  xname=User.IO.Out.ICAConf  xsync=off
  Read CM Dict26 : CarMaker4SL/Read CM Dict  xname=User.IO.Out.AlcSens  xsync=off
  Read CM Dict3 : CarMaker4SL/Read CM Dict  xname=User.IO.Out.MP5_FCWSwitch  xsync=off
  Read CM Dict4 : CarMaker4SL/Read CM Dict  xname=User.IO.Out.MP5_FCW_Sensi  xsync=off
  Read CM Dict5 : CarMaker4SL/Read CM Dict  xname=User.IO.Out.Mp5_ISA_Switch  xsync=off
  Read CM Dict6 : CarMaker4SL/Read CM Dict  xname=User.IO.Out.Mp5_TSR_Switch  xsync=off
  Read CM Dict7 : CarMaker4SL/Read CM Dict  xname=User.IO.Out.Mp5_ISA_Mode  xsync=off
  Read CM Dict8 : CarMaker4SL/Read CM Dict  xname=User.IO.Out.Mp5_LDWWarnMode  xsync=off
  Read CM Dict9 : CarMaker4SL/Read CM Dict  xname=User.IO.Out.MP5_ADAS_SegLmt  xsync=off
  tag scope: MP5_Cmd2Ctrl=global
  wires:
  Read CM Dict/1 -> BusCreator/1  "User.IO.Out.Mp5_LKA_main_SW"
  Read CM Dict1/1 -> BusCreator/2  "User.IO.Out.Mp5_LKA_Mode"
  Read CM Dict2/1 -> BusCreator/3  "User.IO.Out.MP5_AEBSwitch"
  Read CM Dict3/1 -> BusCreator/4  "User.IO.Out.MP5_FCWSwitch"
  Read CM Dict4/1 -> BusCreator/5  "User.IO.Out.MP5_FCW_Sensi"
  Read CM Dict5/1 -> BusCreator/6  "User.IO.Out.Mp5_ISA_Switch"
  Read CM Dict6/1 -> BusCreator/7  "User.IO.Out.Mp5_TSR_Switch"
  Read CM Dict7/1 -> BusCreator/8  "User.IO.Out.Mp5_ISA_Mode"
  Read CM Dict8/1 -> BusCreator/9  "User.IO.Out.Mp5_LDWWarnMode"
  Read CM Dict9/1 -> BusCreator/10  "User.IO.Out.MP5_ADAS_SegLmt"
  Read CM Dict10/1 -> BusCreator/11  "User.IO.Out.MP5_ALCTLC_Mode"
  Read CM Dict11/1 -> BusCreator/12  "User.IO.Out.Mp5_ESA_Cfg"
  Read CM Dict12/1 -> BusCreator/13  "User.IO.Out.Mp5_ELK_Cfg"
  Read CM Dict13/1 -> BusCreator/14  "User.IO.Out.AutoParkingCmd"
  Read CM Dict14/1 -> BusCreator/15  "User.IO.Out.PEPS_RKECommand"
  Read CM Dict15/1 -> BusCreator/16  "User.IO.Out.MP5_BSD_LCW_ACT"
  Read CM Dict22/1 -> BusCreator/17  "User.IO.Out.MP5_FCTA_ACT"
  Read CM Dict16/1 -> BusCreator/18  "User.IO.Out.MP5_RCTA_ACT"
  Read CM Dict17/1 -> BusCreator/19  "User.IO.Out.MP5_DOW_ACT"
  Read CM Dict18/1 -> BusCreator/20  "User.IO.Out.JaBrakConf"
  Read CM Dict19/1 -> BusCreator/21  "User.IO.Out.JaAlertConf"
  Read CM Dict20/1 -> BusCreator/22  "User.IO.Out.JaAlertSens"
  Read CM Dict21/1 -> BusCreator/23  "User.IO.Out.LFConf"
  Read CM Dict23/1 -> BusCreator/24  "User.IO.Out.ICAConf"
  Read CM Dict24/1 -> BusCreator/25  "User.IO.Out.AlcSens"
  Read CM Dict25/1 -> BusCreator/26  "User.IO.Out.ICAConf"
  Read CM Dict26/1 -> BusCreator/27  "User.IO.Out.AlcSens"
  BusCreator/1 -> [MP5_Cmd2Ctrl]

== system MIL4L3_SW6_V1_20220211/CarMaker/VehicleControl/User.IO.Out/SensorStatus2Ctrl ==
  Bus Creator : BusCreator  Inputs=14
  Read CM Dict : CarMaker4SL/Read CM Dict  xname=User.IO.Out.EPS_SteeringTrqS  xsync=off
  Read CM Dict1 : CarMaker4SL/Read CM Dict  xname=User.IO.Out.ESC_ayv_valid  xsync=off
  Read CM Dict10 : CarMaker4SL/Read CM Dict  xname=User.IO.Out.ESC_FRWHeelSpdFlt  xsync=off
  Read CM Dict11 : CarMaker4SL/Read CM Dict  xname=User.IO.Out.ESC_RLWHeelSpdFlt  xsync=off
  Read CM Dict12 : CarMaker4SL/Read CM Dict  xname=User.IO.Out.ESC_RRWHeelSpdFlt  xsync=off
  Read CM Dict13 : CarMaker4SL/Read CM Dict  xname=User.IO.Out.Radar_State  xsync=off
  Read CM Dict2 : CarMaker4SL/Read CM Dict  xname=User.IO.Out.ESC_YawRate_valid  xsync=off
  Read CM Dict3 : CarMaker4SL/Read CM Dict  xname=User.IO.Out.ESC_LonAcc_valid  xsync=off
  Read CM Dict4 : CarMaker4SL/Read CM Dict  xname=User.IO.Out.ESC_VehSpdValid  xsync=off
  Read CM Dict5 : CarMaker4SL/Read CM Dict  xname=User.IO.Out.ESC_FLWHeelPulVal  xsync=off
  Read CM Dict6 : CarMaker4SL/Read CM Dict  xname=User.IO.Out.ESC_FRWHeelPulVal  xsync=off
  Read CM Dict7 : CarMaker4SL/Read CM Dict  xname=User.IO.Out.ESC_RLWHeelPulVal  xsync=off
  Read CM Dict8 : CarMaker4SL/Read CM Dict  xname=User.IO.Out.ESC_RRWHeelPulVal  xsync=off
  Read CM Dict9 : CarMaker4SL/Read CM Dict  xname=User.IO.Out.ESC_FLWHeelSpdFlt  xsync=off
  tag scope: SensorStatus2Ctrl=global
  wires:
  Read CM Dict/1 -> Bus Creator/1  "User.IO.Out.EPS_SteeringTrqS"
  Read CM Dict13/1 -> Bus Creator/14  "User.IO.Out.Radar_State"
  Read CM Dict1/1 -> Bus Creator/2  "User.IO.Out.ESC_ayv_valid"
  Read CM Dict2/1 -> Bus Creator/3  "User.IO.Out.ESC_YawRate_valid"
  Read CM Dict12/1 -> Bus Creator/13  "User.IO.Out.ESC_RRWHeelSpdFlt"
  Read CM Dict3/1 -> Bus Creator/4  "User.IO.Out.ESC_LonAcc_valid"
  Read CM Dict9/1 -> Bus Creator/10  "User.IO.Out.ESC_FLWHeelSpdFlt"
  Read CM Dict10/1 -> Bus Creator/11  "User.IO.Out.ESC_FRWHeelSpdFlt"
  Read CM Dict11/1 -> Bus Creator/12  "User.IO.Out.ESC_RLWHeelSpdFlt"
  Read CM Dict4/1 -> Bus Creator/5  "User.IO.Out.ESC_VehSpdValid"
  Read CM Dict5/1 -> Bus Creator/6  "User.IO.Out.ESC_FLWHeelPulVal"
  Read CM Dict8/1 -> Bus Creator/9  "User.IO.Out.ESC_RRWHeelPulVal"
  Read CM Dict6/1 -> Bus Creator/7  "User.IO.Out.ESC_FRWHeelPulVal"
  Read CM Dict7/1 -> Bus Creator/8  "User.IO.Out.ESC_RLWHeelPulVal"
  Bus Creator/1 -> [SensorStatus2Ctrl]

== system MIL4L3_SW6_V1_20220211/CarMaker/IPG Vehicle/CarAndTrailer/CarAndTrailerUpd/CreateBus Brake.IF.In ==
  In : Inport
  BusCreator : BusCreator  Inputs=9
  Demux : Demux  Outputs=9
  Out : Outport
  wires:
  Demux/9 -> BusCreator/9  "Brake IF Trq_Reg RR"
  Demux/8 -> BusCreator/8  "Brake IF Trq_Reg RL"
  Demux/7 -> BusCreator/7  "Brake IF Trq_Reg FR"
  Demux/6 -> BusCreator/6  "Brake IF Trq_Reg FL"
  Demux/5 -> BusCreator/5  "Brake IF Trq_Reg_max RR"
  Demux/4 -> BusCreator/4  "Brake IF Trq_Reg_max RL"
  Demux/3 -> BusCreator/3  "Brake IF Trq_Reg_max FR"
  Demux/2 -> BusCreator/2  "Brake IF Trq_Reg_max FL"
  Demux/1 -> BusCreator/1  "Brake IF T_env"
  BusCreator/1 -> Out/1
  In/1 -> Demux/1

== system MIL4L3_SW6_V1_20220211/CarMaker/IPG Vehicle/CarAndTrailer/Forces/External Suspension Forces ==
  note: The FSpring/FDamp/FStabi/FBuf outputs of this subsystem will be
      | active if the SuspExtFrcs.Kind entry in the vehicle parameter file
      | is either not present or is empty or has the value "CM4SL".
  note: Insert your suspension forces model here.
  Sync_In : Inport
  lSpring : Inport  Port=2
  vDamp : Inport  Port=3
  lStabi : Inport  Port=4
  lBuf : Inport  Port=5
  Bus Creator{,5..7} (4 alike) : BusCreator  Inputs=8
  Bus Creator{1..4} (4 alike) : BusCreator  Inputs=4
  Demux{1..4} (4 alike) : Demux  Outputs=8
  Ground{,1..15} (16 alike) : Ground
  Terminator{1..4,12} (5 alike) : Terminator
  FSpring : Outport
  FDamp : Outport  Port=2
  FStabi : Outport  Port=3
  FBuf : Outport  Port=4
  wires:
  Bus Creator7/1 -> Terminator4/1
  Bus Creator6/1 -> Terminator3/1
  Bus Creator5/1 -> Terminator2/1
  Bus Creator/1 -> Terminator1/1
  Demux4/8 -> Bus Creator7/8  "vBuf RR"
  Demux4/7 -> Bus Creator7/7  "vBuf RL"
  Demux4/6 -> Bus Creator7/6  "vBuf FR"
  Demux4/5 -> Bus Creator7/5  "vBuf FL"
  Demux3/8 -> Bus Creator6/8  "vStabi RR"
  Demux3/7 -> Bus Creator6/7  "vStabi RL"
  Demux3/6 -> Bus Creator6/6  "vStabi FR"
  Demux3/5 -> Bus Creator6/5  "vStabi FL"
  Demux2/8 -> Bus Creator5/8  "vDamp RR"
  Demux2/7 -> Bus Creator5/7  "vDamp RL"
  Demux2/6 -> Bus Creator5/6  "vDamp FR"
  Demux2/5 -> Bus Creator5/5  "vDamp FL"
  Demux1/8 -> Bus Creator/8  "vSpring RR"
  Demux1/7 -> Bus Creator/7  "vSpring RL"
  Demux1/6 -> Bus Creator/6  "vSpring FR"
  Demux1/5 -> Bus Creator/5  "vSpring FL"
  Demux2/4 -> Bus Creator5/4  "lDamp RR"
  Demux2/3 -> Bus Creator5/3  "lDamp RL"
  Demux2/2 -> Bus Creator5/2  "lDamp FR"
  Demux2/1 -> Bus Creator5/1  "lDamp FL"
  Demux1/4 -> Bus Creator/4  "lSpring RR"
  Demux1/3 -> Bus Creator/3  "lSpring RL"
  Demux1/2 -> Bus Creator/2  "lSpring FR"
  Demux1/1 -> Bus Creator/1  "lSpring FL"
  Demux3/4 -> Bus Creator6/4  "lStabi RR"
  Demux3/3 -> Bus Creator6/3  "lStabi RL"
  Demux3/2 -> Bus Creator6/2  "lStabi FR"
  Demux3/1 -> Bus Creator6/1  "lStabi FL"
  lStabi/1 -> Demux3/1
  vDamp/1 -> Demux2/1
  lSpring/1 -> Demux1/1
  Demux4/4 -> Bus Creator7/4  "lBuf RR"
  Demux4/3 -> Bus Creator7/3  "lBuf RL"
  Demux4/2 -> Bus Creator7/2  "lBuf FR"
  Demux4/1 -> Bus Creator7/1  "lBuf FL"
  lBuf/1 -> Demux4/1
  Ground14/1 -> Bus Creator4/1  "FBuf FL"
  Ground15/1 -> Bus Creator4/2  "FBuf FR"
  Ground12/1 -> Bus Creator4/3  "FBuf RL"
  Ground13/1 -> Bus Creator4/4  "FBuf RR"
  Bus Creator4/1 -> FBuf/1
  Sync_In/1 -> Terminator12/1
  Bus Creator2/1 -> FSpring/1
  Ground/1 -> Bus Creator2/1  "FSpring FL"
  Ground1/1 -> Bus Creator2/2  "FSpring FR"
  Ground2/1 -> Bus Creator2/3  "FSpring RL"
  Ground3/1 -> Bus Creator2/4  "FSpring RR"
  Ground4/1 -> Bus Creator1/1  "FDamp FL"
  Ground5/1 -> Bus Creator1/2  "FDamp FR"
  Ground6/1 -> Bus Creator1/3  "FDamp RL"
  Ground7/1 -> Bus Creator1/4  "FDamp RR"
  Bus Creator1/1 -> FDamp/1
  Ground8/1 -> Bus Creator3/1  "FStabi FL"
  Ground9/1 -> Bus Creator3/2  "FStabi FR"
  Ground10/1 -> Bus Creator3/3  "FStabi RL"
  Ground11/1 -> Bus Creator3/4  "FStabi RR"
  Bus Creator3/1 -> FStabi/1

== system MIL4L3_SW6_V1_20220211/CarMaker/IPG Vehicle/CarAndTrailer/Forces/Tires ==
  note: The TireXX_Out signals will only be used if FileIdent is "CarMaker-Tire-CM4SL" in the tire parameter file!
      | An example parameter file can be found in Data/Tire/DT_CM4SL_UserTire.
  Sync_In : Inport
  TireFL_In : Inport  Port=2
  TireFR_In : Inport  Port=3
  TireRL_In : Inport  Port=4
  TireRR_In : Inport  Port=5
  Bus Creator{1..4} (4 alike) : BusCreator  Inputs=11
  Demux{1..3,8} (4 alike) : Demux  Outputs=7
  TireFL : Subsystem
  TireFR : Subsystem
  TireRL : Subsystem
  TireRR : Subsystem
  TireFL_Out : Outport
  TireFR_Out : Outport  Port=2
  TireRL_Out : Outport  Port=3
  TireRR_Out : Outport  Port=4
  wires:
  Sync_In/1 -> TireRR/1(Sync_In), TireRL/1(Sync_In), TireFR/1(Sync_In), TireFL/1(Sync_In)
  Bus Creator4/1 -> TireRR_Out/1
  Bus Creator2/1 -> TireRL_Out/1
  Bus Creator1/1 -> TireFR_Out/1
  Demux3/5 -> TireRR/6(Rim_turnv)  "Tire_In Rim_turnv"
  Demux3/4 -> TireRR/5(Rim_rotv)  "Tire_In Rim_rotv"
  Demux3/1 -> TireRR/2(Load)  "Tire_In Load"
  Demux3/7 -> TireRR/8(muRoad)  "Tire_In mu"
  Demux3/6 -> TireRR/7(InclinAngle)  "Tire_In Camber"
  Demux3/2 -> TireRR/3(vxtrans)  "Tire_In vxtrans"
  Demux3/3 -> TireRR/4(vytrans)  "Tire_In vytrans"
  TireRR/11(AlignTrq) -> Bus Creator4/11  "Tire_Out AlignTrq"
  TireRR/10(RollResist) -> Bus Creator4/10  "Tire_Out RollResist"
  TireRR/9(OverturnTrq) -> Bus Creator4/9  "Tire_Out OverturnTrq"
  TireRR/8(LoadFrc) -> Bus Creator4/8  "Tire_Out LoadFrc"
  TireRR/7(SideFrc) -> Bus Creator4/7  "Tire_Out SideFrc"
  TireRR/6(LongFrc) -> Bus Creator4/6  "Tire_Out LongFrc"
  TireRR/5(vBelt) -> Bus Creator4/5  "Tire_Out vBelt"
  TireRR/4(rBelt_eff) -> Bus Creator4/4  "Tire_Out rBelt_eff"
  TireRR/3(TurnSlp) -> Bus Creator4/3  "Tire_Out TurnSlp"
  TireRR/1(Slp) -> Bus Creator4/1  "Tire_Out Slp"
  TireRR/2(Alpha) -> Bus Creator4/2  "Tire_Out Alpha"
  Demux2/5 -> TireRL/6(Rim_turnv)  "Tire_In Rim_turnv"
  Demux2/4 -> TireRL/5(Rim_rotv)  "Tire_In Rim_rotv"
  Demux2/1 -> TireRL/2(Load)  "Tire_In Load"
  Demux2/7 -> TireRL/8(muRoad)  "Tire_In mu"
  Demux2/6 -> TireRL/7(InclinAngle)  "Tire_In Camber"
  Demux2/2 -> TireRL/3(vxtrans)  "Tire_In vxtrans"
  Demux2/3 -> TireRL/4(vytrans)  "Tire_In vytrans"
  TireRL/11(AlignTrq) -> Bus Creator2/11  "Tire_Out AlignTrq"
  TireRL/10(RollResist) -> Bus Creator2/10  "Tire_Out RollResist"
  TireRL/9(OverturnTrq) -> Bus Creator2/9  "Tire_Out OverturnTrq"
  TireRL/8(LoadFrc) -> Bus Creator2/8  "Tire_Out LoadFrc"
  TireRL/7(SideFrc) -> Bus Creator2/7  "Tire_Out SideFrc"
  TireRL/6(LongFrc) -> Bus Creator2/6  "Tire_Out LongFrc"
  TireRL/5(vBelt) -> Bus Creator2/5  "Tire_Out vBelt"
  TireRL/4(rBelt_eff) -> Bus Creator2/4  "Tire_Out rBelt_eff"
  TireRL/3(TurnSlp) -> Bus Creator2/3  "Tire_Out TurnSlp"
  TireRL/1(Slp) -> Bus Creator2/1  "Tire_Out Slp"
  TireRL/2(Alpha) -> Bus Creator2/2  "Tire_Out Alpha"
  Demux1/5 -> TireFR/6(Rim_turnv)  "Tire_In Rim_turnv"
  Demux1/4 -> TireFR/5(Rim_rotv)  "Tire_In Rim_rotv"
  Demux1/1 -> TireFR/2(Load)  "Tire_In Load"
  Demux1/7 -> TireFR/8(muRoad)  "Tire_In mu"
  Demux1/6 -> TireFR/7(InclinAngle)  "Tire_In Camber"
  Demux1/2 -> TireFR/3(vxtrans)  "Tire_In vxtrans"
  Demux1/3 -> TireFR/4(vytrans)  "Tire_In vytrans"
  TireFR/11(AlignTrq) -> Bus Creator1/11  "Tire_Out AlignTrq"
  TireFR/10(RollResist) -> Bus Creator1/10  "Tire_Out RollResist"
  TireFR/9(OverturnTrq) -> Bus Creator1/9  "Tire_Out OverturnTrq"
  TireFR/8(LoadFrc) -> Bus Creator1/8  "Tire_Out LoadFrc"
  TireFR/7(SideFrc) -> Bus Creator1/7  "Tire_Out SideFrc"
  TireFR/6(LongFrc) -> Bus Creator1/6  "Tire_Out LongFrc"
  TireFR/5(vBelt) -> Bus Creator1/5  "Tire_Out vBelt"
  TireFR/4(rBelt_eff) -> Bus Creator1/4  "Tire_Out rBelt_eff"
  TireFR/3(TurnSlp) -> Bus Creator1/3  "Tire_Out TurnSlp"
  TireFR/1(Slp) -> Bus Creator1/1  "Tire_Out Slp"
  TireFR/2(Alpha) -> Bus Creator1/2  "Tire_Out Alpha"
  Demux8/5 -> TireFL/6(Rim_turnv)  "Tire_In Rim_turnv"
  Demux8/4 -> TireFL/5(Rim_rotv)  "Tire_In Rim_rotv"
  TireFL_In/1 -> Demux8/1
  Demux8/1 -> TireFL/2(Load)  "Tire_In Load"
  Demux8/7 -> TireFL/8(muRoad)  "Tire_In mu"
  Demux8/6 -> TireFL/7(InclinAngle)  "Tire_In Camber"
  Demux8/2 -> TireFL/3(vxtrans)  "Tire_In vxtrans"
  Demux8/3 -> TireFL/4(vytrans)  "Tire_In vytrans"
  TireFL/11(AlignTrq) -> Bus Creator3/11  "Tire_Out AlignTrq"
  TireFL/10(RollResist) -> Bus Creator3/10  "Tire_Out RollResist"
  TireFL/9(OverturnTrq) -> Bus Creator3/9  "Tire_Out OverturnTrq"
  TireFL/8(LoadFrc) -> Bus Creator3/8  "Tire_Out LoadFrc"
  TireFL/7(SideFrc) -> Bus Creator3/7  "Tire_Out SideFrc"
  TireFL/6(LongFrc) -> Bus Creator3/6  "Tire_Out LongFrc"
  TireFL/5(vBelt) -> Bus Creator3/5  "Tire_Out vBelt"
  TireFL/4(rBelt_eff) -> Bus Creator3/4  "Tire_Out rBelt_eff"
  TireFL/3(TurnSlp) -> Bus Creator3/3  "Tire_Out TurnSlp"
  TireFL/1(Slp) -> Bus Creator3/1  "Tire_Out Slp"
  TireFL/2(Alpha) -> Bus Creator3/2  "Tire_Out Alpha"
  Bus Creator3/1 -> TireFL_Out/1
  TireFR_In/1 -> Demux1/1
  TireRL_In/1 -> Demux2/1
  TireRR_In/1 -> Demux3/1

== system MIL4L3_SW6_V1_20220211/CarMaker/IPG Vehicle/CarAndTrailer/Forces/Vehicle Forces ==
  Sync_In : Inport
  Bus Creator1 : BusCreator  Inputs=12
  Bus Creator8 : BusCreator  Inputs=16
  BusCreator1 : BusCreator  Inputs=4
  BusCreator2 : BusCreator  Inputs=9
  Demux : Demux  Outputs=16
  Demux1 : Demux  Outputs=12
  Demux2 : Demux  Outputs=13
  Forces : S-Function  FunctionName=CM_Sfun  Parameters='Forces'  SFunctionDeploymentMode=off  EnableBusSupport=off
  Terminator : Terminator
  Sync_Out : Outport
  Car.Virtual : Outport  Port=2
  Car.Aero : Outport  Port=3
  Car.Load : Outport  Port=4
  wires:
  BusCreator1/1 -> Terminator/1  "Aero IF (in)"
  Demux2/13 -> BusCreator2/9  "car Aero Trq_1 z"
  Demux2/12 -> BusCreator2/8  "car Aero Trq_1 y"
  Demux2/11 -> BusCreator2/7  "car Aero Trq_1 x"
  Demux2/10 -> BusCreator2/6  "car Aero Frc_1 z"
  Demux2/9 -> BusCreator2/5  "car Aero Frc_1 y"
  Demux2/8 -> BusCreator2/4  "car Aero Frc_1 x"
  Demux2/7 -> BusCreator2/3  "car Aero PoA_1 z"
  Demux2/6 -> BusCreator2/2  "car Aero PoA_1 y"
  Demux2/5 -> BusCreator2/1  "car Aero PoA_1 x"
  Demux2/4 -> BusCreator1/4  "car Aero tau_1"
  Demux2/3 -> BusCreator1/3  "car Aero ApproachVel_1 z"
  Demux2/2 -> BusCreator1/2  "car Aero ApproachVel_1 y"
  Demux2/1 -> BusCreator1/1  "car Aero ApproachVel_1 x"
  Demux/16 -> Bus Creator8/16  "Car Load_3 tz"
  Demux/15 -> Bus Creator8/15  "Car Load_3 ty"
  Demux/14 -> Bus Creator8/14  "Car Load_3 tx"
  Demux/13 -> Bus Creator8/13  "Car Load_3 mass"
  Demux1/12 -> Bus Creator1/12  "Car Virtual Trq_0 z"
  Demux1/11 -> Bus Creator1/11  "Car Virtual Trq_0 y"
  Demux1/10 -> Bus Creator1/10  "Car Virtual Trq_0 x"
  Demux1/9 -> Bus Creator1/9  "Car Virtual Trq_1 z"
  Demux1/8 -> Bus Creator1/8  "Car Virtual Trq_1 y"
  Demux1/7 -> Bus Creator1/7  "Car Virtual Trq_1 x"
  Demux1/6 -> Bus Creator1/6  "Car Virtual Frc_0 z"
  Demux1/5 -> Bus Creator1/5  "Car Virtual Frc_0 y"
  Demux1/4 -> Bus Creator1/4  "Car Virtual Frc_0 x"
  Sync_In/1 -> Forces/1
  Forces/1 -> Sync_Out/1
  BusCreator2/1 -> Car.Aero/1
  Demux1/1 -> Bus Creator1/1  "Car Virtual Frc_1 x"
  Demux1/2 -> Bus Creator1/2  "Car Virtual Frc_1 y"
  Demux1/3 -> Bus Creator1/3  "Car Virtual Frc_1 z"
  Forces/3 -> Demux2/1
  Forces/2 -> Demux1/1
  Bus Creator1/1 -> Car.Virtual/1
  Bus Creator8/1 -> Car.Load/1
  Demux/1 -> Bus Creator8/1  "Car Load_0 mass"
  Demux/2 -> Bus Creator8/2  "Car Load_0 tx"
  Demux/3 -> Bus Creator8/3  "Car Load_0 ty"
  Demux/4 -> Bus Creator8/4  "Car Load_0 tz"
  Demux/5 -> Bus Creator8/5  "Car Load_1 mass"
  Demux/6 -> Bus Creator8/6  "Car Load_1 tx"
  Demux/7 -> Bus Creator8/7  "Car Load_1 ty"
  Demux/8 -> Bus Creator8/8  "Car Load_1 tz"
  Demux/9 -> Bus Creator8/9  "Car Load_2 mass"
  Demux/10 -> Bus Creator8/10  "Car Load_2 tx"
  Demux/11 -> Bus Creator8/11  "Car Load_2 ty"
  Demux/12 -> Bus Creator8/12  "Car Load_2 tz"
  Forces/4 -> Demux/1

== system MIL4L3_SW6_V1_20220211/CarMaker/IPG Vehicle/CarAndTrailer/Trailer/CreateBus Car.Hitch.FrcTrq ==
  In1 : Inport
  Bus Creator7 : BusCreator  Inputs=6
  Demux7 : Demux  Outputs=6
  Out1 : Outport
  wires:
  In1/1 -> Demux7/1
  Bus Creator7/1 -> Out1/1
  Demux7/6 -> Bus Creator7/6  "Car Hitch Trq2Car z"
  Demux7/5 -> Bus Creator7/5  "Car Hitch Trq2Car y"
  Demux7/4 -> Bus Creator7/4  "Car Hitch Trq2Car x"
  Demux7/3 -> Bus Creator7/3  "Car Hitch Frc2Car z"
  Demux7/2 -> Bus Creator7/2  "Car Hitch Frc2Car y"
  Demux7/1 -> Bus Creator7/1  "Car Hitch Frc2Car x"

== system MIL4L3_SW6_V1_20220211/CarMaker/IPG Vehicle/CarAndTrailer/Trailer/CreateBus Vhcl.Motion ==
  In1 : Inport
  BusCreator : BusCreator  Inputs=15
  Demux : Demux  Outputs=15
  Out1 : Outport
  wires:
  Demux/15 -> BusCreator/15  "Vhcl YawAcc"
  Demux/14 -> BusCreator/14  "Vhcl YawVel"
  Demux/13 -> BusCreator/13  "Vhcl Yaw"
  Demux/12 -> BusCreator/12  "Vhcl PitchAcc"
  Demux/11 -> BusCreator/11  "Vhcl PitchVel"
  Demux/10 -> BusCreator/10  "Vhcl Pitch"
  Demux/9 -> BusCreator/9  "Vhcl RollAcc"
  Demux/8 -> BusCreator/8  "Vhcl RollVel"
  Demux/7 -> BusCreator/7  "Vhcl Roll"
  Demux/6 -> BusCreator/6  "Vhcl Hitch_Pos z"
  Demux/5 -> BusCreator/5  "Vhcl Hitch_Pos y"
  Demux/4 -> BusCreator/4  "Vhcl Hitch_Pos x"
  Demux/3 -> BusCreator/3  "Vhcl sRoad"
  Demux/2 -> BusCreator/2  "Vhcl Distance"
  Demux/1 -> BusCreator/1  "Vhcl v"
  In1/1 -> Demux/1
  BusCreator/1 -> Out1/1

== system MIL4L3_SW6_V1_20220211/CarMaker/IPG Vehicle/CarAndTrailer/Trailer/CreateBus Vhcl.PoI ==
  In1 : Inport
  Bus Creator3 : BusCreator  Inputs=18
  Demux3 : Demux  Outputs=18
  Out1 : Outport
  wires:
  Demux3/18 -> Bus Creator3/18  "Vhcl PoI_GCS Elev"
  Demux3/17 -> Bus Creator3/17  "Vhcl PoI_GCS Lat"
  Demux3/16 -> Bus Creator3/16  "Vhcl PoI_GCS Long"
  Demux3/15 -> Bus Creator3/15  "Vhcl PoI_Acc_1 z"
  Demux3/14 -> Bus Creator3/14  "Vhcl PoI_Acc_1 y"
  Demux3/13 -> Bus Creator3/13  "Vhcl PoI_Acc_1 x"
  Demux3/12 -> Bus Creator3/12  "Vhcl PoI_Vel_1 z"
  Demux3/11 -> Bus Creator3/11  "Vhcl PoI_Vel_1 y"
  Demux3/10 -> Bus Creator3/10  "Vhcl PoI_Vel_1 x"
  Demux3/9 -> Bus Creator3/9  "Vhcl PoI_Acc z"
  Demux3/8 -> Bus Creator3/8  "Vhcl PoI_Acc y"
  Demux3/7 -> Bus Creator3/7  "Vhcl PoI_Acc x"
  Demux3/6 -> Bus Creator3/6  "Vhcl PoI_Vel z"
  Demux3/5 -> Bus Creator3/5  "Vhcl PoI_Vel y"
  Demux3/4 -> Bus Creator3/4  "Vhcl PoI_Vel x"
  Demux3/3 -> Bus Creator3/3  "Vhcl PoI_Pos z"
  Demux3/2 -> Bus Creator3/2  "Vhcl PoI_Pos y"
  In1/1 -> Demux3/1
  Bus Creator3/1 -> Out1/1
  Demux3/1 -> Bus Creator3/1  "Vhcl PoI_Pos x"

== system MIL4L3_SW6_V1_20220211/CarMaker/IPG Vehicle/CarAndTrailer/Trailer/CreateBus Vhcl.Steering ==
  In1 : Inport
  Bus Creator3 : BusCreator  Inputs=4
  Demux : Demux
  Out1 : Outport
  wires:
  Bus Creator3/1 -> Out1/1
  Demux/1 -> Bus Creator3/1  "Vhcl Steering Ang"
  Demux/3 -> Bus Creator3/3  "Vhcl Steering AngAcc"
  Demux/2 -> Bus Creator3/2  "Vhcl Steering AngVel"
  Demux/4 -> Bus Creator3/4  "Vhcl Steering Trq"
  In1/1 -> Demux/1

== system MIL4L3_SW6_V1_20220211/CarMaker/IPG Vehicle/CarAndTrailer/Trailer/CreateBus Vhcl.Wheel.FL ==
  In1 : Inport
  Bus Creator3 : BusCreator  Inputs=14
  Demux3 : Demux  Outputs=14
  Out1 : Outport
  wires:
  Demux3/14 -> Bus Creator3/14  "Vhcl Wheel FL Trq_WhlBearing"
  Demux3/13 -> Bus Creator3/13  "Vhcl Wheel FL Trq_T2W"
  Demux3/12 -> Bus Creator3/12  "Vhcl Wheel FL SideSlip"
  Demux3/11 -> Bus Creator3/11  "Vhcl Wheel FL LongSlip"
  Demux3/10 -> Bus Creator3/10  "Vhcl Wheel FL vBelt"
  Demux3/9 -> Bus Creator3/9  "Vhcl Wheel FL Fz"
  Demux3/8 -> Bus Creator3/8  "Vhcl Wheel FL Fy"
  Demux3/7 -> Bus Creator3/7  "Vhcl Wheel FL Fx"
  Demux3/6 -> Bus Creator3/6  "Vhcl Wheel FL r_zxy z"
  Demux3/5 -> Bus Creator3/5  "Vhcl Wheel FL r_zxy y"
  Demux3/4 -> Bus Creator3/4  "Vhcl Wheel FL r_zxy x"
  Demux3/3 -> Bus Creator3/3  "Vhcl Wheel FL t z"
  Demux3/2 -> Bus Creator3/2  "Vhcl Wheel FL t y"
  In1/1 -> Demux3/1
  Bus Creator3/1 -> Out1/1
  Demux3/1 -> Bus Creator3/1  "Vhcl Wheel FL t x"

== system MIL4L3_SW6_V1_20220211/CarMaker/IPG Vehicle/CarAndTrailer/Trailer/CreateBus Vhcl.Wheel.FR ==
  In1 : Inport
  Bus Creator3 : BusCreator  Inputs=14
  Demux3 : Demux  Outputs=14
  Out1 : Outport
  wires:
  Demux3/14 -> Bus Creator3/14  "Vhcl Wheel FR Trq_WhlBearing"
  Demux3/13 -> Bus Creator3/13  "Vhcl Wheel FR Trq_T2W"
  Demux3/12 -> Bus Creator3/12  "Vhcl Wheel FR SideSlip"
  Demux3/11 -> Bus Creator3/11  "Vhcl Wheel FR LongSlip"
  Demux3/10 -> Bus Creator3/10  "Vhcl Wheel FR vBelt"
  Demux3/9 -> Bus Creator3/9  "Vhcl Wheel FR Fz"
  Demux3/8 -> Bus Creator3/8  "Vhcl Wheel FR Fy"
  Demux3/7 -> Bus Creator3/7  "Vhcl Wheel FR Fx"
  Demux3/6 -> Bus Creator3/6  "Vhcl Wheel FR r_zxy z"
  Demux3/5 -> Bus Creator3/5  "Vhcl Wheel FR r_zxy y"
  Demux3/4 -> Bus Creator3/4  "Vhcl Wheel FR r_zxy x"
  Demux3/3 -> Bus Creator3/3  "Vhcl Wheel FR t z"
  Demux3/2 -> Bus Creator3/2  "Vhcl Wheel FR t y"
  In1/1 -> Demux3/1
  Bus Creator3/1 -> Out1/1
  Demux3/1 -> Bus Creator3/1  "Vhcl Wheel FR t x"

== system MIL4L3_SW6_V1_20220211/CarMaker/IPG Vehicle/CarAndTrailer/Trailer/CreateBus Vhcl.Wheel.RL ==
  In1 : Inport
  Bus Creator3 : BusCreator  Inputs=14
  Demux3 : Demux  Outputs=14
  Out1 : Outport
  wires:
  Demux3/14 -> Bus Creator3/14  "Vhcl Wheel RL Trq_WhlBearing"
  Demux3/13 -> Bus Creator3/13  "Vhcl Wheel RL Trq_T2W"
  Demux3/12 -> Bus Creator3/12  "Vhcl Wheel RL SideSlip"
  Demux3/11 -> Bus Creator3/11  "Vhcl Wheel RL LongSlip"
  Demux3/10 -> Bus Creator3/10  "Vhcl Wheel RL vBelt"
  Demux3/9 -> Bus Creator3/9  "Vhcl Wheel RL Fz"
  Demux3/8 -> Bus Creator3/8  "Vhcl Wheel RL Fy"
  Demux3/7 -> Bus Creator3/7  "Vhcl Wheel RL Fx"
  Demux3/6 -> Bus Creator3/6  "Vhcl Wheel RL r_zxy z"
  Demux3/5 -> Bus Creator3/5  "Vhcl Wheel RL r_zxy y"
  Demux3/4 -> Bus Creator3/4  "Vhcl Wheel RL r_zxy x"
  Demux3/3 -> Bus Creator3/3  "Vhcl Wheel RL t z"
  Demux3/2 -> Bus Creator3/2  "Vhcl Wheel RL t y"
  In1/1 -> Demux3/1
  Bus Creator3/1 -> Out1/1
  Demux3/1 -> Bus Creator3/1  "Vhcl Wheel RL t x"
